simulink subsystem "OnlineID"  (R2021a)
settings: Solver=VariableStepAuto  StartTime=0.0  StopTime=10.0  RelTol=1e-3
(part 2 of 2)

== stateflow chart OnlineID/OnlineID ==
  settings: updateMethod=DISCRETE  sampleTime=1/d_f_states
  note: Online identification
      | of flux maps and linear pmsm parameters
  state OnlineIDSuperState
    entry:
    InitParams;
    enteredOnlineID=boolean(1);
    OnlineID_output.activeState=uint16(500);
    during:
    state RefreshDataRegister
      entry:
      OnlineID_output.activeState=uint16(501);
      counter=uint32(1);
      omega_register=single(zeros(5,1));
      id_register=single(zeros(50,1));
      iq_register=single(zeros(50,1));
      vd_register=single(zeros(50,1));
      vq_register=single(zeros(50,1));
      iq_const=boolean(0);
      id_const=boolean(0);
      omega_const=boolean(0);
      breakback=single(0);
      during:
      counter=uint32(counter+1);
      counter_time=uint32(counter_time+1);
      iq_sum=iq_sum+single(ActualValues.i_dq.q);
      id_sum=id_sum+single(ActualValues.i_dq.d);
      vd_sum=vd_sum+single(ActualValues.v_dq.d);
      vq_sum=vq_sum+single(ActualValues.v_dq.q);
      omega_sum=omega_sum+single(ActualValues.omega_m);
      if(mod(counter,uint32(0.01/GlobalConfig.sampleTimeISR))==0)
      RefreshDataRegister;
      iq_register(1,1)=iq_sum/(0.01/GlobalConfig.sampleTimeISR);
      id_register(1,1)=id_sum/(0.01/GlobalConfig.sampleTimeISR);
      vd_register(1,1)=vd_sum/(0.01/GlobalConfig.sampleTimeISR);
      vq_register(1,1)=vq_sum/(0.01/GlobalConfig.sampleTimeISR);
      iq_sum=single(0);
      id_sum=single(0);
      vd_sum=single(0);
      vq_sum=single(0);
      if(mod(counter,uint32(0.1/GlobalConfig.sampleTimeISR))==0)
      omega_register(1,1)=omega_sum/(0.1/GlobalConfig.sampleTimeISR);
      omega_sum=single(0);
      [allow_meas,omega_const,iq_const,id_const,i_valid]=CheckSteadyState(abs(iq_register),abs(id_register),abs(omega_register),counter_time);
      end
      end
    state TempPsiCalcState
      entry:
      OnlineID_output.activeState=uint16(504);
      temp_diff=abs(OnlineID_output.Wtemp-OnlineIDConfig.Temp_ref);
      delta_psi=abs(OnlineID_output.psi_pm_out-GlobalConfig.PMSM_config.Psi_PM_Vs);
      if(temp_diff>0&&temp_diff<99)
      OnlineID_output.delta_psi(1+floor(temp_diff),2)= OnlineID_output.delta_psi(1+floor(temp_diff),2)+1;
      OnlineID_output.delta_psi(1+floor(temp_diff),1)= OnlineID_output.delta_psi(1+floor(temp_diff),1)+delta_psi;
      end
      breakback=single(2);
    state PsiCalcState
      entry:
      OnlineID_output.activeState=uint16(503);
      Wtemp_check=((single(OnlineID_output.Rph_out)/single(GlobalConfig.PMSM_config.R_ph_Ohm))-single(1))*....
      single(254.453)+single(OnlineIDConfig.Temp_ref);
      if(Wtemp_check<200&&Wtemp_check>(-100))
      OnlineID_output.Wtemp =Wtemp_check;
      end
      if(OnlineIDConfig.array_cleaned==1)
      OnlineID_output.psi_array=cleaned_psi_array;
      OnlineID_output.clean_array = boolean(0);
      end
      array_counter=uint16(99);
      psi_d=1000*(mean(vq_register)-OnlineID_output.Rph_out*mean(iq_register))/(mean(omega_register)*GlobalConfig.PMSM_config.polePairs);
      psi_q=1000*(-1)*(mean(vd_register)-OnlineID_output.Rph_out*mean(id_register))/(mean(omega_register)*GlobalConfig.PMSM_config.polePairs);
      OnlineID_output.psi_array(1,array_counter)=mean(id_register);
      OnlineID_output.psi_array(2,array_counter)=mean(iq_register);
      OnlineID_output.psi_array(3,array_counter)=mean(omega_register);
      OnlineID_output.psi_array(4,array_counter)=OnlineID_output.Wtemp;
      OnlineID_output.psi_array(5,array_counter)=psi_d;
      OnlineID_output.psi_array(6,array_counter)=psi_q;
      OnlineID_output.clean_array=boolean(1);
      breakback=single(1);
    state CalcLinearParamsState
      entry:
      OnlineID_output.activeState = uint16(502);
      OnlineID_output.IdControlFlag=boolean(1);
      iq1counter=single(0);
      iq2counter=single(0);
      id1counter=single(0);
      id2counter=single(0);
      Vd1counter=single(0);
      Vd2counter=single(0);
      Vq1counter=single(0);
      Vq2counter=single(0);
      omega1counter=single(0);
      omega2counter=single(0);
      stop_ident=boolean(0);
      omega_sum=single(0);
      iq_sum=single(0);
      counter=uint32(1);
      if((counter_time>=(uint32(OnlineIDConfig.Rs_time/GlobalConfig.sampleTimeISR))) && (i_valid==0))  %Sets variable to 1, if Rs will be identified
      LinPara_ident_outside=boolean(1);                      % outside the valid range
      else
      LinPara_ident_outside=boolean(0);
      end
      if(i_valid==1)
      counter_time=uint32(0);    %Resets the timer, since the lin.Para. will be identified
      end                                        %inside the valid range
      omega_register_alt=omega_register;
      id_register_alt=id_register;
      iq_register_alt=iq_register; %uses the old values of State501 as starting point
      omega_register_neu=single(zeros(5,1));
      id_register_neu=single(zeros(10,1));
      iq_register_neu=single(zeros(10,1));
      during:
      OnlineID_output.id_out=i_d_R_online;
      counter=counter+uint32(1);
      identParams;
      iq_sum=iq_sum+single(ActualValues.i_dq.q);
      id_sum=id_sum+single(ActualValues.i_dq.d);
      omega_sum=omega_sum+single(ActualValues.omega_m); %averages iq over 100 and omega over 200 measuring points
      if(mod(counter,uint32(0.01/GlobalConfig.sampleTimeISR))==0)
      RefreshDataRegister;
      iq_register_neu(1,1)=iq_sum/(0.01/GlobalConfig.sampleTimeISR);
      id_register_neu(1,1)=id_sum/(0.01/GlobalConfig.sampleTimeISR);
      iq_sum=single(0);
      id_sum=single(0);
      if(mod(counter,uint32(0.02/GlobalConfig.sampleTimeISR))==0)
      omega_register_neu(1,1)=omega_sum/(0.02/GlobalConfig.sampleTimeISR);
      omega_sum=single(0);
      end
      if(mod(counter,uint32(0.1/GlobalConfig.sampleTimeISR))==0)%checks every 0.1s if current omega and iq is too different from the old one
      [stop_ident] = Break(abs(iq_register_alt),abs(id_register_alt),abs(omega_register_alt),abs(iq_register_neu),abs(id_register_neu),abs(omega_register_neu));
      end
      end
      exit:
      OnlineID_output.id_out=single(0.0);
      OnlineID_output.IdControlFlag=boolean(0);
    (default) -> OnlineIDSuperState.RefreshDataRegister
    TempPsiCalcState -> OnlineIDSuperState.RefreshDataRegister : [breakback==2]
    OnlineIDSuperState.RefreshDataRegister -> PsiCalcState [order 2] : [LinPara_ident_outside==0 && OnlineIDConfig.allowPsiCalcOutside==0 ....
        | && allow_meas==0&&omega_const==1&&iq_const==1]
    PsiCalcState -> TempPsiCalcState : [breakback==1]
    OnlineIDSuperState.RefreshDataRegister -> CalcLinearParamsState [order 1] : [allow_meas==1&&omega_const==1....
        | &&iq_const==1&&id_const==1]
    CalcLinearParamsState -> OnlineIDSuperState.RefreshDataRegister [order 1] : [stop_ident==1]
    CalcLinearParamsState -> OnlineIDSuperState.RefreshDataRegister [order 3] : [OnlineIDConfig.allowPsiCalcOutside==0 && LinPara_ident_outside==1....
        |  && counter==uint32((1.2/GlobalConfig.sampleTimeISR)+1)]
    OnlineIDSuperState.RefreshDataRegister -> PsiCalcState [order 3] : [OnlineIDConfig.allowPsiCalcOutside==1 ....
        | && allow_meas==0&&omega_const==1&&iq_const==1]
    CalcLinearParamsState -> PsiCalcState [order 2] : [OnlineIDConfig.allowPsiCalcOutside==1 && counter==uint32((1.2/GlobalConfig.sampleTimeISR)+1)....
        |  || LinPara_ident_outside==0 && OnlineIDConfig.allowPsiCalcOutside==0 &&....
        |  counter==uint32((1.2/GlobalConfig.sampleTimeISR)+1)]
  state Waiting
    entry:
    %wait for activation of
    %OnlineID
    %donothing
  note: ---
  note: Philipp Gebhardt, October 2019:
      |
      | Description of OnlineID Stateflow:
      |
      | This Stateflow is used to detect special transient states and to gather measuring data in these states.The measuremen data is stored in arrays which are transmitted to other functions thate are called in main.c to keep the isr.c as clean and small as possible.
      | For more information of the identification methods see documentation in the project reports and the master thesis.
      |
      | The description is structured in the differrent states which are numbered by the active State variable.
      |
      | OnlineIDSuperState-activeState#500
      |
      | When entering this State all local and output Variables are intialized by calling the function "InitParams".
      | During the SuperState it is searched for the "FluxUpdatedFlag", in order to reset the "UpdateFluxFlag" which is used for triggering the flux maps calculation.
      | Furthermore, it is searched for the "ResetOnlineFlag" to reset all local and output variables if requested.
      | OnlineIDSuperState is always carried out (always active). While entering OnlineIDSuperState the "RefreshDataRegister" state is entered as well.
      |
      | RefreshDataRegisterState-activeState#501
      |
      | In this state a shifting data register of iq-current, id-current, ud-voltage, uq-voltage and of speed is filled with measuring values.This register is used to detect special states as acceleration or steady state.
      | Therefore, the data register is updated in a specific time interval with averaged measuring values, which are determined by sum up the measurements with a counter and multiplied afterwards with the inverse factor of the measurment-number (e.g. 0.01).
      | Considering the different time constants of current and speed, there are different time intervals beeing observed.
      | In case of the current signal, there are 100 measuring values averaged. In case of the speed signal, there are 1000 measuring values averaged.
      | As a result of this, as well as to consider the same time period, there are 50 current values in the data register and 5 speed values.
      | In every iteration the data register is checked, if there is a special state like acceleration or steady state.
      | If there is acceleration, the inertia identification is performed. (Caution this identification is not experienced on hardware)
      | If steady state is identified and the machine is in its valid range, all the other parameter identification states are performed and "CalcLinearParamsState" is entered.
      | If only steady state is detected, "CalcLinearParamsState" will not be entered and the next state will be "PsiCalcState".
      | If the machine operates outside its valid range for an extended period of time, a identification outside of the nominal range will be performed. This means, if "counter_time" exceeds a set time, "CalcLinearParamsState" will be entered, even if the machine is not in its valid range.
      | If "allowPsiCalcOutside" is set to 0 (default), the flux maps will only be calculated with the linear parameters, which have been identified inside the valid range. If it is set to 1, the flux map will be always calculated, even if the linear parameters have been identified outside the valide range.
      |
      | CalcLinearParamsState-activeState#502
      |
      | In this state a d-current rectangular signal is injected, while recording the d-q-voltages, the d-q-currents and omega.
      | During the injection phase the dq-currents and the speed will be monitored and stored in a data-register. If the difference between the average value of these data registers and the average of the data registers in State501 exceeds a threshold, the injection phase
      | will be aborted. This way the influence of sudden changes in the speed or torque of the machine on the identification processes can be avoided. After the injection phase is aborted, State501 will be entered again.
      | In assistance of the function call "identParams" the linear machine parameters are calculated form the recorded values.
      | If the linear Parameters have been identified inside the valid range, state 503 will always be entered after this state.
      | If the linear Parameters have been identified outside the valid range, state 503 will only be entered, if "allowPsiCalcOutside"==1. Otherwise state 501 will be entered again.
      | The State can only be entered if there is an Inputflag "allowStepFlag" which allows the d-current-step, if the flag is denied during the state, the state is canceled and "RefreshDataRegisterState" is entered again.
      | If the d-current step is accomplished, the "PsiCalsState" is entered.
      |
      | PsiCalcState-activeState#503
      |
      | In this state the winding temperature is calculated based on the difference between online identified phase resistance and the reference resitance value, which is given by the input "Rph_in" as well as its reference temperature by the input "Temp_ref".
      | Therefore, the specific resistance temperature dependency of copper needs to be considered with the factor 254.453 K/ohm [Hoerner].
      | After the plausibility of the winding temperature is checked, the flux values for generating the flux maps are calculated from the measuring data stored in the data register.
      | If there is a new array that was cleaned in the main, "array_cleaned_flag" is true and the cleaned array is copied in the output array before the new measurement values are stored in the output array. This ensures no lose of measuring data through cleaning the array.
      | After the new array values are added, the "clean_array_flag" signalizes the "CleanPsiArray" function (in the main.c) that there is a new demand for cleaning the array.
      |
      | TempPsiCalcState-activeState#504
      |
      | In this state the measurement data for the calculation of the temperature dependency of the permantent flux is written into the "delta_psi_array" which is then evaluated by a regression-line in the "InterpolationMeshGrid" function (in the main.c).
      | Thererfore, the differences to the reference values of psi_PM and the temperature are calculated. To save RAM the regression-line function uses the floored temperature difference as array index. To increase the
      | accuracy of the regression, the flux difference values are averaged about a high amount of samples through summing up the measuring data and a counter in the second array column. So before evaluation, the array real values need to be
      | calcualated by a division of column 1 through column 2.
      | After this state "RefreshDataRegisterState" is entered again.
  Waiting -> OnlineIDSuperState : [ControlFlags.enableOnlineID==1 && GlobalConfig.Reset==0....
      | && OnlineIDConfig.OnlineID_Reset==0 &&....
      |  ControlFlags.finished_all_Offline_states==1]
  (default) -> Waiting
  OnlineIDSuperState -> Waiting : [ControlFlags.enableOnlineID==0 || GlobalConfig.Reset==1 ||....
      |  OnlineIDConfig.OnlineID_Reset==1 || GlobalConfig.enableParameterID==0]
      | {InitParams;enteredOnlineID=boolean(0)}
  data: allow_measurement function_output; om_con function_output; iq_con function_output; id_con function_output; iq_reg_in function_input; id_reg_in function_input; om_reg_in function_input; i_val function_output; timer function_input; stop_identParams function_output; iq_reg_alt function_input; id_reg_alt function_input; om_reg_alt function_input; iq_reg_neu function_input; id_reg_neu function_input; om_reg_neu function_input; breakback local; accel local; array_counter local; counter local; i_d_R_online local; omega_sum local; id_sum local; iq_sum local; vq_sum local; vd_sum local; Wtemp_check local; id1counter local; id2counter local; iq1counter local; iq2counter local; omega1counter local; omega2counter local; Vd1counter local; Vd2counter local; Vq1counter local; Vq2counter local; temp_diff local; delta_psi local; R_old local; R_veryold local; PsiPm_old local; PsiPm_veryold local; Ld_old local; Ld_veryold local; Lq_old local; Lq_veryold local; cleaned_psi_array input size=[6,100]; omega_register local; omega_const local; iq_const local; vd_register local; vq_register local; id_register local; iq_register local; id_const local; counter_time local; allow_meas local; i_valid local; LinPara_ident_outside local; stop_ident local; iq_register_alt local; iq_register_neu local; omega_register_alt local; omega_register_neu local; id_register_alt local; id_register_neu local; counter_ausserhalb local; R_old_outside local; R_veryold_outside local; counter_innerhalb local; Ld_veryold_outside local; Ld_old_outside local; Lq_veryold_outside local; Lq_old_outside local; PsiPm_veryold_outside local; PsiPm_old_outside local; OnlineIDConfig input Bus: uz_ParaID_OnlineIDConfig_t; ActualValues input Bus: uz_ParaID_ActualValues_t; GlobalConfig input Bus: uz_ParaID_GlobalConfig_t; ControlFlags input Bus: uz_ParaID_ControlFlags_t; psi_d local; psi_q local; psi_temp_const local; UpdateFluxFlag local; OnlineID_output output Bus: uz_ParaID_OnlineID_output_t; enteredOnlineID output
  function [allow_measurement, om_con,iq_con,id_con,i_val]=CheckSteadyState(iq_reg_in,id_reg_in,om_reg_in,timer):
    | function [allow_measurement, om_con,iq_con,id_con,i_val]=CheckSteadyState(iq_reg_in,id_reg_in,om_reg_in,timer)
    | 
    | mean_om_reg=mean(om_reg_in);
    | mean_id_reg=mean(id_reg_in);
    | mean_iq_reg=mean(iq_reg_in);
    | 
    | if((mean_iq_reg+(OnlineIDConfig.dev_curr*GlobalConfig.ratCurrent))>=max(iq_reg_in)...
    |         &&(mean_iq_reg-(OnlineIDConfig.dev_curr*GlobalConfig.ratCurrent))<=min(iq_reg_in)&&min(iq_reg_in)~=0)    
    |     iq_con=boolean(1);
    | else
    |     iq_con=boolean(0);
    | end
    | 
    | if((mean_id_reg+(OnlineIDConfig.dev_curr*GlobalConfig.ratCurrent))>=max(id_reg_in)...
    |         &&(mean_id_reg-(OnlineIDConfig.dev_curr*GlobalConfig.ratCurrent))<=min(id_reg_in)&&min(id_reg_in)~=0)    
    |     id_con=boolean(1);    
    | else
    |     id_con=boolean(0);
    | end
    | 
    | if(mean_om_reg<((GlobalConfig.ratSpeed*OnlineIDConfig.max_n_ratio*2*pi)/60) && mean_om_reg>((GlobalConfig.ratSpeed*OnlineIDConfig.min_n_ratio*2*pi)/60))%Drehzahlgrenzwerte in rad/sec
    | if((mean_om_reg+((OnlineIDConfig.dev_omega*GlobalConfig.ratSpeed*2*pi)/60))>=max(om_reg_in)...
    |         &&(mean_om_reg-((OnlineIDConfig.dev_omega*GlobalConfig.ratSpeed*2*pi)/60))<=min(om_reg_in)&&min(om_reg_in)~=0)   
    |     om_con=boolean(1);    
    | else
    |     om_con=boolean(0);
    | end
    | else
    |     om_con=boolean(0);
    | end
    | 
    | if(sqrt(mean_iq_reg^2 + mean_id_reg^2)<OnlineIDConfig.nom_factor*GlobalConfig.ratCurrent)                                 
    |     i_val=boolean(1);             %Checks, if iq- and id-currents are within
    | else                             %the set limit. The variable nom-factor sets 
    |     i_val=boolean(0);             %the range of the allowed limit,  i.e. 
    | end                              %nominal current or 0.5*nominal current
    |                                  %If currents are inside this limit, the 
    |                                  %linear parameters will be measured
    |                                  
    | if((timer >= uint32(OnlineIDConfig.Rs_time*(1/GlobalConfig.sampleTimeISR))) && i_val==0)  %Rs_time in seconds 
    |     allow_measurement = boolean(1);  %If the machine operates for a set time outside
    | elseif(i_val==1)                    %the current limit, the measurement of the linear
    |     allow_measurement = boolean(1);  %parameter start again regardless of the machine state
    | else
    |     allow_measurement = boolean(0);
    | end    
    | end
  function RefreshDataRegister:
    | function RefreshDataRegister
    | 
    | if(mod(counter,uint32(0.1/GlobalConfig.sampleTimeISR))==0)
    |     m=length(omega_register);
    |     for k= uint16(0):uint16(m-2)
    |         omega_register(m-k)=omega_register(m-(k+1));
    |     end
    | end
    |  m=length(iq_register);
    |  for k= uint16(0):uint16(m-2)
    |    iq_register(m-k)=iq_register(m-(k+1));
    |    id_register(m-k)=id_register(m-(k+1));
    |    vd_register(m-k)=vd_register(m-(k+1));
    |    vq_register(m-k)=vq_register(m-(k+1));
    | end
    |  
    | end
  function identParams:
    | function identParams 
    | 
    |    % positive halfperiod
    |    if(counter <= uint32(0.6/GlobalConfig.sampleTimeISR))
    |             i_d_R_online = single(+OnlineIDConfig.identRAmp);
    |             if(counter >= uint32((0.5/GlobalConfig.sampleTimeISR)-1) && counter < uint32((0.6/GlobalConfig.sampleTimeISR)-1))
    |                 Vd1counter = Vd1counter+ActualValues.v_dq.d;
    |                 Vq1counter = Vq1counter+ActualValues.v_dq.q;
    |                 id1counter = id1counter+ActualValues.i_dq.d;
    |                 iq1counter = iq1counter+ActualValues.i_dq.q;               
    |                 omega1counter = omega1counter+ActualValues.omega_el;
    |             end
    |    end
    |     
    |    % negative halfperiod       
    |    if(counter > uint32(0.6/GlobalConfig.sampleTimeISR) && counter < uint32(1.2/GlobalConfig.sampleTimeISR))
    |             i_d_R_online = single(-OnlineIDConfig.identRAmp);
    |             if(counter >= uint32((1.1/GlobalConfig.sampleTimeISR)-1) && counter < uint32((1.2/GlobalConfig.sampleTimeISR)-1))
    |                 Vd2counter = Vd2counter+ActualValues.v_dq.d;
    |                 Vq2counter = Vq2counter+ActualValues.v_dq.q;
    |                 id2counter = id2counter+ActualValues.i_dq.d;
    |                 iq2counter = iq2counter+ActualValues.i_dq.q;
    |                 omega2counter= omega2counter+ActualValues.omega_el;
    |             end
    |    end
    |         
    |    %    Averaging    halfperiods
    |    if(counter == uint32(1.2/GlobalConfig.sampleTimeISR))
    |                 Vq1counter=Vq1counter/(0.1/GlobalConfig.sampleTimeISR);
    |                 Vq2counter=Vq2counter/(0.1/GlobalConfig.sampleTimeISR);
    |                 Vd1counter=Vd1counter/(0.1/GlobalConfig.sampleTimeISR);
    |                 Vd2counter=Vd2counter/(0.1/GlobalConfig.sampleTimeISR);
    |                 id1counter=id1counter/(0.1/GlobalConfig.sampleTimeISR);
    |                 id2counter=id2counter/(0.1/GlobalConfig.sampleTimeISR);
    |                 iq1counter=iq1counter/(0.1/GlobalConfig.sampleTimeISR);
    |                 iq2counter=iq2counter/(0.1/GlobalConfig.sampleTimeISR);
    |                 omega1counter=omega1counter/(0.1/GlobalConfig.sampleTimeISR);
    |                 omega2counter=omega2counter/(0.1/GlobalConfig.sampleTimeISR);
    |                 
    |     %Calculation of Parameters            
    | 
    |                 %     Calculate R              
    |                         R_check= single(  ( Vd2counter/ (iq2counter*omega2counter) -  Vd1counter/(iq1counter*omega1counter)  )  /...
    |                         (  id2counter/(iq2counter* omega2counter) -   id1counter/ (iq1counter*omega1counter)       )       );
    |                     
    |   
    |                 %     Simplification for small reluctance torque: iq1 ~ iq2 ~ (iq1+iq2)/2 ; omega1~omega2~(omega1+omega2)/2
    |    
    |                
    |                 %     Calculate Lq 
    |                         Lq_check=single(Vd1counter*id2counter-Vd2counter*id1counter)/(omega2counter*iq2counter*id1counter-omega1counter*iq1counter*id2counter);  
    |                                      
    |                 %     Calculate permanent flux 
    |                          psipm_check=single((Vq1counter-R_check*iq1counter)*id2counter)/(omega1counter*(id2counter-id1counter))-...
    |                             ((Vq2counter-R_check*iq2counter)*id1counter)/(omega2counter*(id2counter-id1counter));
    |                     
    |                 %     Calculate Ld 
    |                          Ld_check=single((Vq2counter-Vq1counter)-(iq2counter-iq1counter)*R_check - psipm_check*(omega2counter - omega1counter))/...
    |                          (id2counter*omega2counter-id1counter*omega1counter); 
    |                  
    |                  
    |                 %     Plausibilty Checks          
    |                          if(Ld_check>0&&Ld_check<1)
    |                             if(OnlineIDConfig.AverageTransParams==1)
    | 								 if(LinPara_ident_outside==1 && counter_ausserhalb==1)
    |                                    %Average over 3 iterations
    | 									Ld_veryold_outside=Ld_old_outside;
    | 									Ld_old_outside=OnlineID_output.Ld_out;
    | 									OnlineID_output.Ld_out=(Ld_check+Ld_old_outside+Ld_veryold_outside)/single(3.0);
    | 								elseif(LinPara_ident_outside==1 && counter_ausserhalb==0)
    | 									Ld_veryold_outside=Ld_old;
    | 									Ld_old_outside=OnlineID_output.Ld_out;
    | 									OnlineID_output.Ld_out=(Ld_check+Ld_old_outside+Ld_veryold_outside)/single(3.0);
    | 								end
    | 								if(LinPara_ident_outside==0 && counter_innerhalb==1)
    | 									Ld_veryold=Ld_old;
    |                                     Ld_old=OnlineID_output.Ld_out;
    |                                     OnlineID_output.Ld_out=(Ld_check+Ld_old+Ld_veryold)/single(3.0);
    | 								elseif(LinPara_ident_outside==0 && counter_innerhalb==0)
    | 									OnlineID_output.Ld_out=(Ld_check+Ld_old+Ld_veryold)/single(3.0);
    | 								end
    |                             else
    |                                 OnlineID_output.Ld_out=Ld_check;
    |                             end
    |                          end
    |              
    |                          if(Lq_check>0&&Lq_check<1)
    |                             if(OnlineIDConfig.AverageTransParams==1)
    | 								 if(LinPara_ident_outside==1 && counter_ausserhalb==1)
    |                                    %Average over 3 iterations
    | 									Lq_veryold_outside=Lq_old_outside;
    | 									Lq_old_outside=OnlineID_output.Lq_out;
    | 									OnlineID_output.Lq_out=(Lq_check+Lq_old_outside+Lq_veryold_outside)/single(3.0);
    | 								elseif(LinPara_ident_outside==1 && counter_ausserhalb==0)
    | 									Lq_veryold_outside=Lq_old;
    | 									Lq_old_outside=OnlineID_output.Lq_out;
    | 									OnlineID_output.Lq_out=(Lq_check+Lq_old_outside+Lq_veryold_outside)/single(3.0);
    | 								end
    | 								if(LinPara_ident_outside==0 && counter_innerhalb==1)
    | 									Lq_veryold=Lq_old;
    |                                     Lq_old=OnlineID_output.Lq_out;
    |                                     OnlineID_output.Lq_out=(Lq_check+Lq_old+Lq_veryold)/single(3.0);
    | 								elseif(LinPara_ident_outside==0 && counter_innerhalb==0)
    | 									OnlineID_output.Lq_out=(Lq_check+Lq_old+Lq_veryold)/single(3.0);
    | 								end
    |                             else
    |                                 OnlineID_output.Lq_out=Lq_check;
    |                             end
    |                          end
    |                 
    |                         if(psipm_check>0&&psipm_check<1)
    |                             if(OnlineIDConfig.AverageTransParams==1)
    | 									if(LinPara_ident_outside==1 && counter_ausserhalb==1)
    | 										%Average over 3 iterations
    | 										PsiPm_veryold_outside=PsiPm_old_outside;
    | 										PsiPm_old_outside=OnlineID_output.psi_pm_out;
    | 										OnlineID_output.psi_pm_out=(psipm_check+PsiPm_old_outside+PsiPm_veryold_outside)/single(3.0);								
    | 									elseif(LinPara_ident_outside==1 && counter_ausserhalb==0)
    | 										PsiPm_veryold_outside=PsiPm_old;
    | 										PsiPm_old_outside=OnlineID_output.psi_pm_out;
    | 										OnlineID_output.psi_pm_out=(psipm_check+PsiPm_old_outside+PsiPm_veryold_outside)/single(3.0);		
    | 									end								
    | 									if(LinPara_ident_outside==0 && counter_innerhalb==1)
    | 										%Average over 3 iterations
    | 										PsiPm_veryold=PsiPm_old;
    | 										PsiPm_old=OnlineID_output.psi_pm_out;
    | 										OnlineID_output.psi_pm_out=(psipm_check+PsiPm_old+PsiPm_veryold)/single(3.0);								
    | 									elseif(LinPara_ident_outside==0 && counter_innerhalb==0)
    | 										OnlineID_output.psi_pm_out=(psipm_check+PsiPm_old+PsiPm_veryold)/single(3.0);
    | 									end
    |                             else
    |                                 OnlineID_output.psi_pm_out=psipm_check;
    |                             end
    |                         end
    |                 
    |                         if(R_check>0&&R_check<1000)
    |                             if(OnlineIDConfig.AverageTransParams==1)
    | 									if(LinPara_ident_outside==1 && counter_ausserhalb==1)
    | 										%Average over 3 iterations
    | 										R_veryold_outside=R_old_outside;
    | 										R_old_outside=OnlineID_output.Rph_out;
    | 										OnlineID_output.Rph_out=(R_check+R_old_outside+R_veryold_outside)/single(3.0);									
    | 									elseif(LinPara_ident_outside==1 && counter_ausserhalb==0)
    | 										R_veryold_outside=R_old;
    | 										R_old_outside=OnlineID_output.Rph_out;
    | 										OnlineID_output.Rph_out=(R_check+R_old_outside+R_veryold_outside)/single(3.0);
    | 									end								
    | 									if(LinPara_ident_outside==0 && counter_innerhalb==1)
    | 										%Average over 3 iterations
    | 										R_veryold=R_old;
    | 										R_old=OnlineID_output.Rph_out;
    | 										OnlineID_output.Rph_out=(R_check+R_old+R_veryold)/single(3.0);										
    | 									elseif(LinPara_ident_outside==0 && counter_innerhalb==0)
    | 										OnlineID_output.Rph_out=(R_check+R_old+R_veryold)/single(3.0);
    | 									end
    |                             else
    |                                 OnlineID_output.Rph_out=R_check;
    |                              end
    |                         end
    |                         
    | 						if(LinPara_ident_outside==0)%Resets the counter for outside_identification and sets the counter for inside_identification
    | 							counter_ausserhalb=uint16(0);
    | 							counter_innerhalb=uint16(1);
    | 						elseif(LinPara_ident_outside==1)%Resets the counter for inside_identification and sets the counter for outside_identification
    | 							counter_ausserhalb=uint16(1);
    | 							counter_innerhalb=uint16(0);
    | 						end
    |             %   Reset d-current
    |             i_d_R_online = single(0);
    |      end
    |        
    | 
    | end
  function RefreshDataRegister:
    | function RefreshDataRegister
    | 
    | if(mod(counter,uint32(0.02/GlobalConfig.sampleTimeISR))==0)
    |     m=length(omega_register_neu);
    |     for k= uint16(0):uint16(m-2)
    |         omega_register_neu(m-k)=omega_register_neu(m-(k+1));
    |     end
    | end
    |  m=length(iq_register_neu);
    |  for k= uint16(0):uint16(m-2)
    |     iq_register_neu(m-k)=iq_register_neu(m-(k+1));
    |  end
    |  
    |  m=length(id_register_neu);
    |  for k= uint16(0):uint16(m-2)
    |     id_register_neu(m-k)=id_register_neu(m-(k+1));
    |  end
    | 
    | end
  function stop_identParams  = Break(iq_reg_alt,id_reg_alt,om_reg_alt,iq_reg_neu,id_reg_neu,om_reg_neu):
    | function stop_identParams  = Break(iq_reg_alt,id_reg_alt,om_reg_alt,iq_reg_neu,id_reg_neu,om_reg_neu)
    | 
    | %calculates the mean of the registers of the new and old values
    | mean_om_alt=mean(om_reg_alt);%Mittelwert
    | mean_iq_alt=mean(iq_reg_alt);
    | mean_id_alt=mean(id_reg_alt);
    | mean_om_neu=mean(om_reg_neu);
    | mean_iq_neu=mean(iq_reg_neu);
    | mean_id_neu=mean(id_reg_neu);
    | %compares if the new mean iq value is inside the tolerance range of the old
    | %one
    | if((mean_iq_alt+(OnlineIDConfig.dev_curr*GlobalConfig.ratCurrent))>=mean_iq_neu && ...
    |         (mean_iq_alt-(OnlineIDConfig.dev_curr*GlobalConfig.ratCurrent))<= mean_iq_neu)   
    |     iq_break=boolean(0);   
    | else
    |     iq_break=boolean(1);
    | end
    | %compares if the new mean iq value is inside the tolerance range of the old
    | %one
    | if((mean_om_alt+((OnlineIDConfig.dev_omega*GlobalConfig.ratSpeed*2*pi)/60))>=mean_om_neu&&...
    |         (mean_om_alt-((OnlineIDConfig.dev_omega*GlobalConfig.ratSpeed*2*pi)/60))<=mean_om_neu)    
    |     om_break=boolean(0);  
    | else
    |     om_break=boolean(1);
    | end
    | 
    | %compares if the new mean id value is inside the tolerance range of the old
    | %one. Though here the tolerance is bigger than the peak of the id-Step 
    | if((OnlineIDConfig.identRAmp+mean_id_alt+(OnlineIDConfig.dev_curr*GlobalConfig.ratCurrent))>=mean_id_neu&&...
    |         (-OnlineIDConfig.identRAmp+mean_id_alt-(OnlineIDConfig.dev_curr*GlobalConfig.ratCurrent))<=mean_id_neu)    
    |     id_break=boolean(0);  
    | else
    |     id_break=boolean(1);
    | end
    | 
    | %if either the iq or omega increased too much, it will set the value to 1
    | if( om_break == 1 || iq_break == 1 || id_break == 1) 
    |     stop_identParams = boolean(1);
    | else
    |     stop_identParams = boolean(0);
    | end
    | end
  function InitParams:
    | function InitParams
    | 
    | %Steady State Detection
    | vd_sum                              = single(0);
    | vq_sum                              = single(0);
    | id_sum                              = single(0);
    | iq_sum                              = single(0);
    | omega_sum                           = single(0);
    | id_register                         = single(zeros(50,1));
    | iq_register                         = single(zeros(50,1));
    | vd_register                         = single(zeros(50,1));
    | vq_register                         = single(zeros(50,1));
    | id_const                            = boolean(0);
    | iq_const                            = boolean(0);
    | omega_const                         = boolean(0);
    | 
    | %Calculation if linearParams will be identified
    | allow_meas                          = boolean(0);
    | counter_time                        = uint32(0);
    | LinPara_ident_outside               = boolean(1);
    | i_valid                             = boolean(0);
    | counter_ausserhalb                  = uint16(0);
    | counter_innerhalb                   = uint16(0);
    | 
    | 
    | iq1counter                          = single(0);
    | iq2counter                          = single(0);
    | id1counter                          = single(0);
    | id2counter                          = single(0);
    | Vd1counter                          = single(0);
    | Vd2counter                          = single(0);
    | omega1counter                       = single(0);
    | omega2counter                       = single(0);
    | omega_register                      = single(zeros(5,1));
    | 
    | 
    | %Psi Calculation
    | array_counter                       = uint16(1);
    | psi_d                               = single(0);
    | psi_q                               = single(0);
    | R_old                               = single(GlobalConfig.PMSM_config.R_ph_Ohm);
    | R_veryold                           = single(GlobalConfig.PMSM_config.R_ph_Ohm);
    | %%%
    | R_old_outside                       = single(GlobalConfig.PMSM_config.R_ph_Ohm);
    | R_veryold_outside                   = single(GlobalConfig.PMSM_config.R_ph_Ohm);
    | Ld_veryold_outside                  = single(GlobalConfig.PMSM_config.Psi_PM_Vs);
    | Ld_old_outside                      = single(GlobalConfig.PMSM_config.Ld_Henry);
    | Lq_veryold_outside                  = single(GlobalConfig.PMSM_config.Lq_Henry);
    | Lq_old_outside                      = single(GlobalConfig.PMSM_config.Lq_Henry);
    | PsiPm_veryold_outside               = single(GlobalConfig.PMSM_config.Psi_PM_Vs);
    | PsiPm_old_outside                   = single(GlobalConfig.PMSM_config.Psi_PM_Vs);
    | %%%
    | accel                               = single(0);
    | i_d_R_online                        = single(0);
    | UpdateFluxFlag                      = boolean(0);
    | psi_temp_const                      = single(0.0000001);
    | Wtemp_check                         = single(0);
    | PsiPm_old                           = single(GlobalConfig.PMSM_config.Psi_PM_Vs);
    | PsiPm_veryold                       = single(GlobalConfig.PMSM_config.Psi_PM_Vs);
    | Ld_old                              = single(GlobalConfig.PMSM_config.Ld_Henry);
    | Ld_veryold                          = single(GlobalConfig.PMSM_config.Ld_Henry);
    | Lq_old                              = single(GlobalConfig.PMSM_config.Lq_Henry);
    | Lq_veryold                          = single(GlobalConfig.PMSM_config.Lq_Henry);
    | 
    | %Outputs
    | enteredOnlineID=boolean(0);
    | OnlineID_output.id_out              = single(0.0);
    | OnlineID_output.Rph_out             = single(GlobalConfig.PMSM_config.R_ph_Ohm);
    | OnlineID_output.Wtemp               = single(20.0);
    | OnlineID_output.psi_array           = single(zeros(6,100));
    | OnlineID_output.IdControlFlag       = boolean(0);
    | OnlineID_output.delta_psi           = single(zeros(100,2));
    | OnlineID_output.delta_psi(7,1)      = 0.07;
    | OnlineID_output.delta_psi(7,2)      = 1;
    | OnlineID_output.delta_psi(9,1)      = 0.09;
    | OnlineID_output.delta_psi(9,2)      = 1;
    | OnlineID_output.activeState         = uint16(0);
    | OnlineID_output.psi_pm_out          = single(GlobalConfig.PMSM_config.Psi_PM_Vs);
    | OnlineID_output.Ld_out              = single(GlobalConfig.PMSM_config.Ld_Henry);
    | OnlineID_output.Lq_out              = single(GlobalConfig.PMSM_config.Lq_Henry);
    | OnlineID_output.clean_array         = boolean(0);
    | 
    | OnlineID_output.psi_array(1,array_counter)=single(0.70*GlobalConfig.ratCurrent);
    | OnlineID_output.psi_array(2,array_counter)=single(0.7*GlobalConfig.ratCurrent);
    | OnlineID_output.psi_array(3,array_counter)=single(50);
    | OnlineID_output.psi_array(4,array_counter)=OnlineIDConfig.Temp_ref;
    | OnlineID_output.psi_array(5,array_counter)=single(1000*(0.7*GlobalConfig.ratCurrent*GlobalConfig.PMSM_config.Ld_Henry+GlobalConfig.PMSM_config.Psi_PM_Vs));
    | OnlineID_output.psi_array(6,array_counter)=single(1000*(0.7*GlobalConfig.ratCurrent*GlobalConfig.PMSM_config.Lq_Henry));
    | array_counter=array_counter+1;
    | OnlineID_output.psi_array(1,array_counter)=single(-0.75*GlobalConfig.ratCurrent);
    | OnlineID_output.psi_array(2,array_counter)=single(0.75*GlobalConfig.ratCurrent);
    | OnlineID_output.psi_array(3,array_counter)=single(50);
    | OnlineID_output.psi_array(4,array_counter)=OnlineIDConfig.Temp_ref;
    | OnlineID_output.psi_array(5,array_counter)=single(1000*(-0.75*GlobalConfig.ratCurrent*GlobalConfig.PMSM_config.Ld_Henry+GlobalConfig.PMSM_config.Psi_PM_Vs));
    | OnlineID_output.psi_array(6,array_counter)=single(1000*(0.75*GlobalConfig.ratCurrent*GlobalConfig.PMSM_config.Lq_Henry));
    | array_counter=array_counter+1;
    | OnlineID_output.psi_array(1,array_counter)=single(-0.65*GlobalConfig.ratCurrent);
    | OnlineID_output.psi_array(2,array_counter)=single(-0.65*GlobalConfig.ratCurrent);
    | OnlineID_output.psi_array(3,array_counter)=single(50);
    | OnlineID_output.psi_array(4,array_counter)=OnlineIDConfig.Temp_ref;
    | OnlineID_output.psi_array(5,array_counter)=single(1000*(-0.65*GlobalConfig.ratCurrent*GlobalConfig.PMSM_config.Ld_Henry+GlobalConfig.PMSM_config.Psi_PM_Vs));
    | OnlineID_output.psi_array(6,array_counter)=single(1000*(-0.65*GlobalConfig.ratCurrent*GlobalConfig.PMSM_config.Lq_Henry));
    | array_counter=array_counter+1;
    | OnlineID_output.psi_array(1,array_counter)=single(0.6*GlobalConfig.ratCurrent);
    | OnlineID_output.psi_array(2,array_counter)=single(-0.6*GlobalConfig.ratCurrent);
    | OnlineID_output.psi_array(3,array_counter)=single(50);
    | OnlineID_output.psi_array(4,array_counter)=OnlineIDConfig.Temp_ref;
    | OnlineID_output.psi_array(5,array_counter)=single(1000*(0.6*GlobalConfig.ratCurrent*GlobalConfig.PMSM_config.Ld_Henry+GlobalConfig.PMSM_config.Psi_PM_Vs));
    | OnlineID_output.psi_array(6,array_counter)=single(1000*(-0.6*GlobalConfig.ratCurrent*GlobalConfig.PMSM_config.Lq_Henry));
    | array_counter=array_counter+1;
    | % 
    | OnlineID_output.psi_array(1,array_counter)=single(0.30*GlobalConfig.ratCurrent);
    | OnlineID_output.psi_array(2,array_counter)=single(0.3*GlobalConfig.ratCurrent);
    | OnlineID_output.psi_array(3,array_counter)=single(50);
    | OnlineID_output.psi_array(4,array_counter)=OnlineIDConfig.Temp_ref;
    | OnlineID_output.psi_array(5,array_counter)=single(0.3*GlobalConfig.ratCurrent*GlobalConfig.PMSM_config.Ld_Henry+GlobalConfig.PMSM_config.Psi_PM_Vs)*1000;
    | OnlineID_output.psi_array(6,array_counter)=single(0.3*GlobalConfig.ratCurrent*GlobalConfig.PMSM_config.Lq_Henry)*1000;
    | array_counter=array_counter+1;
    | OnlineID_output.psi_array(1,array_counter)=single(-0.35*GlobalConfig.ratCurrent);
    | OnlineID_output.psi_array(2,array_counter)=single(0.35*GlobalConfig.ratCurrent);
    | OnlineID_output.psi_array(3,array_counter)=single(50);
    | OnlineID_output.psi_array(4,array_counter)=OnlineIDConfig.Temp_ref;
    | OnlineID_output.psi_array(5,array_counter)=single(-0.35*GlobalConfig.ratCurrent*GlobalConfig.PMSM_config.Ld_Henry+GlobalConfig.PMSM_config.Psi_PM_Vs)*1000;
    | OnlineID_output.psi_array(6,array_counter)=single(0.35*GlobalConfig.ratCurrent*GlobalConfig.PMSM_config.Lq_Henry)*1000;
    | array_counter=array_counter+1;
    | OnlineID_output.psi_array(1,array_counter)=single(-0.25*GlobalConfig.ratCurrent);
    | OnlineID_output.psi_array(2,array_counter)=single(-0.25*GlobalConfig.ratCurrent);
    | OnlineID_output.psi_array(3,array_counter)=single(50);
    | OnlineID_output.psi_array(4,array_counter)=OnlineIDConfig.Temp_ref;
    | OnlineID_output.psi_array(5,array_counter)=single(-0.25*GlobalConfig.ratCurrent*GlobalConfig.PMSM_config.Ld_Henry+GlobalConfig.PMSM_config.Psi_PM_Vs)*1000;
    | OnlineID_output.psi_array(6,array_counter)=single(-0.25*GlobalConfig.ratCurrent*GlobalConfig.PMSM_config.Lq_Henry)*1000;
    | array_counter=array_counter+1;
    | OnlineID_output.psi_array(1,array_counter)=single(0.2*GlobalConfig.ratCurrent);
    | OnlineID_output.psi_array(2,array_counter)=single(-0.2*GlobalConfig.ratCurrent);
    | OnlineID_output.psi_array(3,array_counter)=single(50);
    | OnlineID_output.psi_array(4,array_counter)=OnlineIDConfig.Temp_ref;
    | OnlineID_output.psi_array(5,array_counter)=single(0.2*GlobalConfig.ratCurrent*GlobalConfig.PMSM_config.Ld_Henry+GlobalConfig.PMSM_config.Psi_PM_Vs)*1000;
    | OnlineID_output.psi_array(6,array_counter)=single(-0.2*GlobalConfig.ratCurrent*GlobalConfig.PMSM_config.Lq_Henry)*1000;
    | array_counter=array_counter+1;
